simulink model "Model_FC_v4"  (R2015a)
settings: Solver=ode3  StartTime=0.0  StopTime=50  FixedStep=0.01  RelTol=1e-3
undefined symbols (not defined in the file): sigbuilder_block
libraries: powerlib x5, simulink x2
settings Model: Creator=Mina  LastModifiedBy=Mina
settings OptimizationCC: BlockReduction=off  ConditionallyExecuteInputs=off

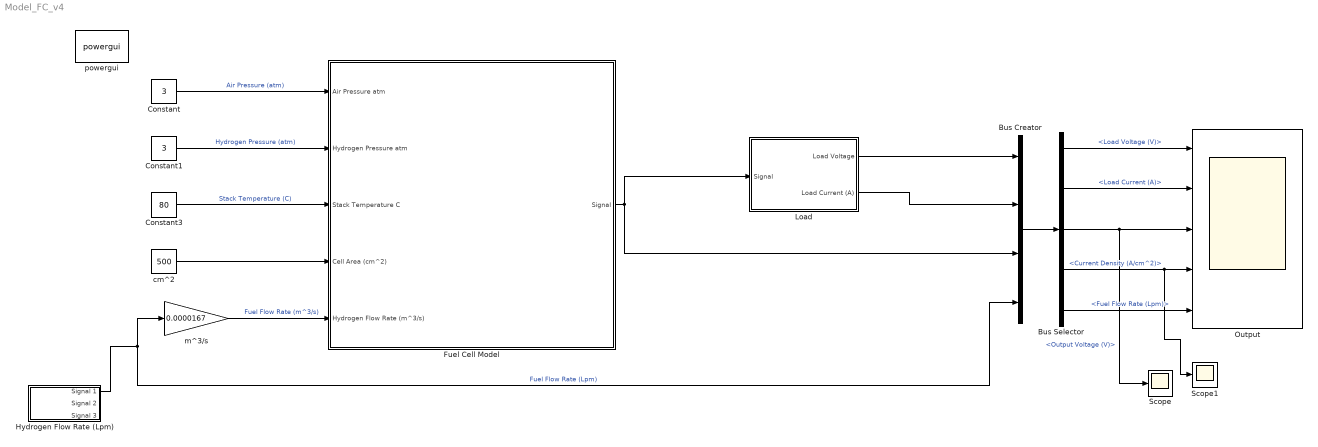
== system Model_FC_v4 ==
  Bus Creator : BusCreator
  Bus Selector : BusSelector  OutputSignals=Load Voltage (V),Load Current (A),signal3.Output Voltage (V),signal3.Current Density (A/cm^2),Fuel Flow Rate (Lpm)
  Constant : Constant  Value=3
  Constant1 : Constant  Value=3
  Constant3 : Constant  Value=80
  Fuel Cell Model : Subsystem
  Hydrogen Flow Rate (Lpm) : Subsystem  Tag=STV Subsys  LoadFcn=sigbuilder_block('load');  StartFcn=sigbuilder_block('start');  StopFcn=sigbuilder_block('stop');  ClipboardFcn=sigbuilder_block('clipboard');  mask(Sigbuilder block){}
      mask help: Simulink:masks:SigbuilderBlock_MD
      mask init:
      | if ~strcmp(get_param(bdroot(gcbh),'SimulationStatus'),'stopped') tuvar = sigbuilder_block('maskInit'); end
      settings: CopyFcn=sigbuilder_block('copy');  DeleteFcn=sigbuilder_block('delete');  ModelCloseFcn=sigbuilder_block('modelClose');  PreSaveFcn=sigbuilder_block('preSave');  PauseFcn=sigbuilder_block('pause');  ContinueFcn=sigbuilder_block('continue');  NameChangeFcn=sigbuilder_block('namechange');  OpenFcn=sigbuilder_block('open',[437.6 199.2 550.4 400 ]);  CloseFcn=sigbuilder_block('close');
      mask Display: plot(0, 0, 100, 100,[2, 2, 32, 32, 2], [68, 8, 8, 68, 68],[32, 2], [38, 38], [32, 19, 2],[53, 60, 44], [32, 17, 17, 2],[16, 16, 31, 31]);txt = getActiveGroup(gcbh);text(2, 100, txt,'verticalAlignment', 'top');
  Load : Subsystem
  "Output " : Scope  NumInputPorts=5
      settings: YMin=6~0.3~0.4~0.8~2.5  YMax=11~0.575~0.8~1.35~4  SaveName=Output_Data
  Scope : Scope
      settings: YMin=0.433555  YMax=0.433555  SaveName=ScopeData3
  Scope1 : Scope
      settings: YMin=1.24134  YMax=1.372  SaveName=ScopeData4
  cm^2 : Constant  Value=500
  m^3/s : Gain  Gain=0.0000167
  powergui : powerlib/powergui  Priority=1  SimulationMode=Continuous  SolverType=Tustin/Backward Euler (TBE)  SampleTime=50e-6  frequency=60  SPID=off  DisableSnubberDevices=off  DisableRonSwitches=off  DisableVfSwitches=off  SwTol=0  DisplayEquations=off  Interpol=off  methode=off  Ts=100  FunctionMessages=off  echomessages=off  HookPort=off  EnableUseOfTLC=off  x0status=blocks  frequencyindice=0  Pbase=100e6  ErrMax=1e-4  Iterations=50  UnitsV=kV  UnitsW=MW  buscounter=0  RestoreLinks=warning  ResistiveCurrentMeasurement=off  Frange=[0:2:500]  Ylog=off  Xlog=on  ShowGrid=off  save=off  variable=ZData  structure=0  ZoomFFT=off  StartTime=0.0  cycles=1  DisplayStyle=1  fundamental=60  FreqAxis=off  MaxFrequency=1000  frequencyindicesteady=1  RmsSteady=1  display=off
  wires:
  Constant3/1 -> Fuel Cell Model/3(Stack Temperature C)  "Stack Temperature (C)"
  cm^2/1 -> Fuel Cell Model/4(Cell Area (cm^2))
  Constant/1 -> Fuel Cell Model/1(Air Pressure atm)  "Air Pressure (atm)"
  Bus Creator/1 -> Bus Selector/1
  Bus Selector/1 -> "Output "/1  "<Load Voltage (V)>"
  Bus Selector/2 -> "Output "/2  "<Load Current (A)>"
  Bus Selector/4 -> Scope1/1, "Output "/4  "<Current Density (A/cm^2)>"
  Constant1/1 -> Fuel Cell Model/2(Hydrogen Pressure atm)  "Hydrogen Pressure (atm)"
  m^3/s/1 -> Fuel Cell Model/5(Hydrogen Flow Rate (m^3/s))  "Fuel Flow Rate (m^3/s)"
  Fuel Cell Model/1(Signal) -> Load/1(Signal), Bus Creator/3
  Bus Selector/3 -> Scope/1, "Output "/3  "<Output Voltage (V)>"
  Load/2(Load Current (A)) -> Bus Creator/2
  Load/1(Load Voltage) -> Bus Creator/1
  Hydrogen Flow Rate (Lpm)/1(Signal 1) -> Bus Creator/4, m^3/s/1  "Fuel Flow Rate (Lpm)"
  Bus Selector/5 -> "Output "/5  "<Fuel Flow Rate (Lpm)>"

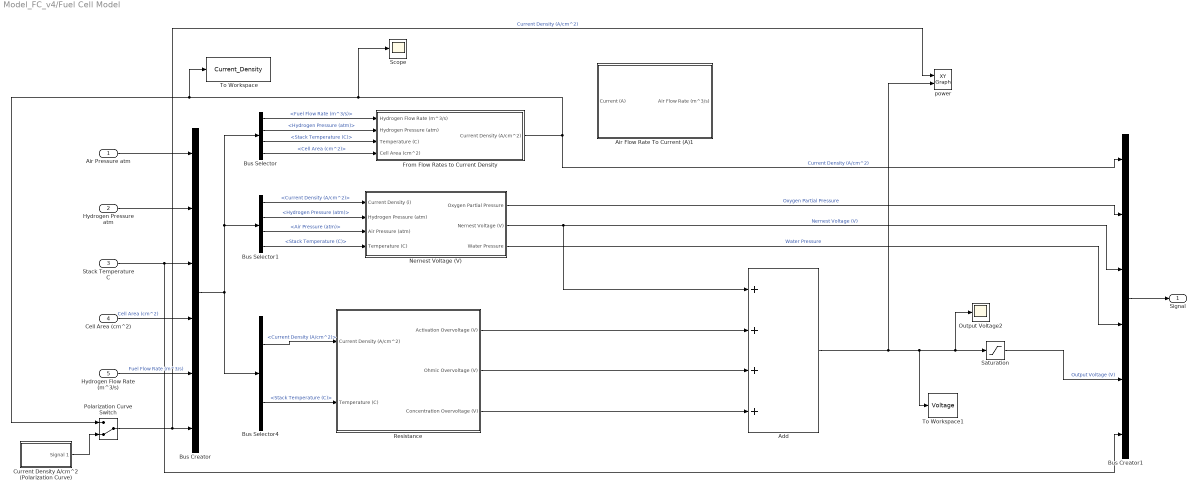
== system Model_FC_v4/Fuel Cell Model ==
  Air Pressure atm : Inport
  Hydrogen Pressure atm : Inport  Port=2
  Stack Temperature C : Inport  Port=3
  Cell Area (cm^2) : Inport  Port=4
  Hydrogen Flow Rate (m^3/s) : Inport  Port=5
  Add : Sum  Inputs=++++
  Air Flow Rate To Current (A)1 : Subsystem
  Bus Creator : BusCreator  Inputs=6
  Bus Creator1 : BusCreator  Inputs=6
  Bus Selector : BusSelector  OutputSignals=Fuel Flow Rate (m^3/s),Hydrogen Pressure (atm),Stack Temperature (C),Cell Area (cm^2)
  Bus Selector1 : BusSelector  OutputSignals=Current Density (A/cm^2),Hydrogen Pressure (atm),Air Pressure (atm),Stack Temperature (C)
  Bus Selector4 : BusSelector  OutputSignals=Current Density (A/cm^2),Stack Temperature (C)
  Current Density A/cm^2 (Polarization Curve) : Subsystem  Tag=STV Subsys  LoadFcn=sigbuilder_block('load');  StartFcn=sigbuilder_block('start');  StopFcn=sigbuilder_block('stop');  ClipboardFcn=sigbuilder_block('clipboard');  mask(Sigbuilder block){}
      mask help: Simulink:masks:SigbuilderBlock_MD
      mask init:
      | if ~strcmp(get_param(bdroot(gcbh),'SimulationStatus'),'stopped') tuvar = sigbuilder_block('maskInit'); end
      settings: CopyFcn=sigbuilder_block('copy');  DeleteFcn=sigbuilder_block('delete');  ModelCloseFcn=sigbuilder_block('modelClose');  PreSaveFcn=sigbuilder_block('preSave');  PauseFcn=sigbuilder_block('pause');  ContinueFcn=sigbuilder_block('continue');  NameChangeFcn=sigbuilder_block('namechange');  OpenFcn=sigbuilder_block('open',[437.6 199.2 550.4 400 ]);  CloseFcn=sigbuilder_block('close');
      mask Display: plot(0, 0, 100, 100,[2, 2, 32, 32, 2], [68, 8, 8, 68, 68],[32, 2], [38, 38], [32, 19, 2],[53, 60, 44], [32, 17, 17, 2],[16, 16, 31, 31]);txt = getActiveGroup(gcbh);text(2, 100, txt,'verticalAlignment', 'top');
  From Flow Rates to Current Density : Subsystem
  Nernest Voltage (V) : Subsystem
  Output Voltage2 : Scope
      settings: YMin=0.941209  YMax=0.941209  Decimation=2
  Polarization Curve Switch : ManualSwitch  CurrentSetting=0
  Resistance : Subsystem
  Saturation : Saturate  UpperLimit=inf  LowerLimit=0
  Scope : Scope
      settings: YMin=1.63334  YMax=1.63334
  To Workspace : ToWorkspace  VariableName=Current_Density  SampleTime=-1
      settings: Save2DSignal=2-D array (concatenate along first dimension)
  To Workspace1 : ToWorkspace  VariableName=Voltage  SampleTime=-1
      settings: Save2DSignal=2-D array (concatenate along first dimension)
  power : simulink/Sinks/XY Graph  xmin=0  xmax=1.5  ymin=0.0  ymax=1.4  st=0
  Signal : Outport
  wires:
  Add/1 -> power/2, To Workspace1/1, Output Voltage2/1, Saturation/1
  Cell Area (cm^2)/1 -> Bus Creator/4  "Cell Area (cm^2)"
  Saturation/1 -> Bus Creator1/5  "Output Voltage (V)"
  Current Density A/cm^2 (Polarization Curve)/1(Signal 1) -> Polarization Curve Switch/2
  Air Pressure atm/1 -> Bus Creator/1
  Hydrogen Pressure atm/1 -> Bus Creator/2
  Stack Temperature C/1 -> Bus Creator1/6, Bus Creator/3
  Hydrogen Flow Rate (m^3/s)/1 -> Bus Creator/5  "Fuel Flow Rate (m^3/s)"
  Bus Creator/1 -> Bus Selector1/1, Bus Selector/1, Bus Selector4/1
  From Flow Rates to Current Density/1(Current Density (A/cm^2)) -> Scope/1, To Workspace/1, Polarization Curve Switch/1, Bus Creator1/1  "Current Density (A/cm^2)"
  Bus Selector/1 -> From Flow Rates to Current Density/1(Hydrogen Flow Rate (m^3/s))  "<Fuel Flow Rate (m^3/s)>"
  Bus Selector/2 -> From Flow Rates to Current Density/2(Hydrogen Pressure (atm))  "<Hydrogen Pressure (atm)>"
  Bus Selector/3 -> From Flow Rates to Current Density/3(Temperature (C))  "<Stack Temperature (C)>"
  Bus Selector/4 -> From Flow Rates to Current Density/4(Cell Area (cm^2))  "<Cell Area (cm^2)>"
  Nernest Voltage (V)/2(Nernest Voltage (V)) -> Bus Creator1/3, Add/1  "Nernest Voltage (V)"
  Bus Selector1/1 -> Nernest Voltage (V)/1(Current Density (i))  "<Current Density (A/cm^2)>"
  Bus Selector1/2 -> Nernest Voltage (V)/2(Hydrogen Pressure (atm))  "<Hydrogen Pressure (atm)>"
  Bus Selector1/3 -> Nernest Voltage (V)/3(Air Pressure (atm))  "<Air Pressure (atm)>"
  Bus Selector1/4 -> Nernest Voltage (V)/4(Temperature (C))  "<Stack Temperature (C)>"
  Nernest Voltage (V)/1(Oxygen Partial Pressure) -> Bus Creator1/2  "Oxygen Partial Pressure"
  Nernest Voltage (V)/3(Water Pressure) -> Bus Creator1/4  "Water Pressure"
  Bus Selector4/1 -> Resistance/1(Current Density (A/cm^2))  "<Current Density (A/cm^2)>"
  Bus Selector4/2 -> Resistance/2(Temperature (C))  "<Stack Temperature (C)>"
  Resistance/1(Activation Overvoltage (V)) -> Add/2
  Resistance/2(Ohmic Overvoltage (V)) -> Add/3
  Resistance/3(Concentration Overvoltage (V)) -> Add/4
  Polarization Curve Switch/1 -> power/1, Bus Creator/6  "Current Density (A/cm^2)"
  Bus Creator1/1 -> Signal/1

== system Model_FC_v4/Hydrogen Flow Rate (Lpm) ==
  Demux : Demux  Tag=STV Demux  Outputs=3
  FromWs : FromWorkspace  Tag=STV FromWs  VariableName=tuvar  SampleTime=0
      SigBuilderData=|
      | common.afterFinalStr = 'Extrapolate'
      | common.sampleTime = 0
      | dataSet.timeRange = [0 10]
      | dataSet.name = 'Group 1'
      | sbobj.Groups.Name = 'Group 1'
      | sbobj.Groups.Signals(1).Name = 'Signal 1'
      | sbobj.Groups.Signals(1).XData = [0 5 7.5 10]
      | sbobj.Groups.Signals(1).YData = [2.5 2.5 4 4]
      | sbobj.Groups.Signals(2).Name = 'Signal 2'
      | sbobj.Groups.Signals(2).XData = [0 5 5 10]
      | sbobj.Groups.Signals(2).YData = [2.5 2.5 4 4]
      | sbobj.Groups.Signals(3).Name = 'Signal 3'
      | sbobj.Groups.Signals(3).XData = [0 10]
      | sbobj.Groups.Signals(3).YData = [4 4]
  Signal 1 : Outport  Tag=STV Outport
  Signal 2 : Outport  Tag=STV Outport  Port=2
  Signal 3 : Outport  Tag=STV Outport  Port=3
  wires:
  Demux/1 -> Signal 1/1
  FromWs/1 -> Demux/1
  Demux/2 -> Signal 2/1
  Demux/3 -> Signal 3/1

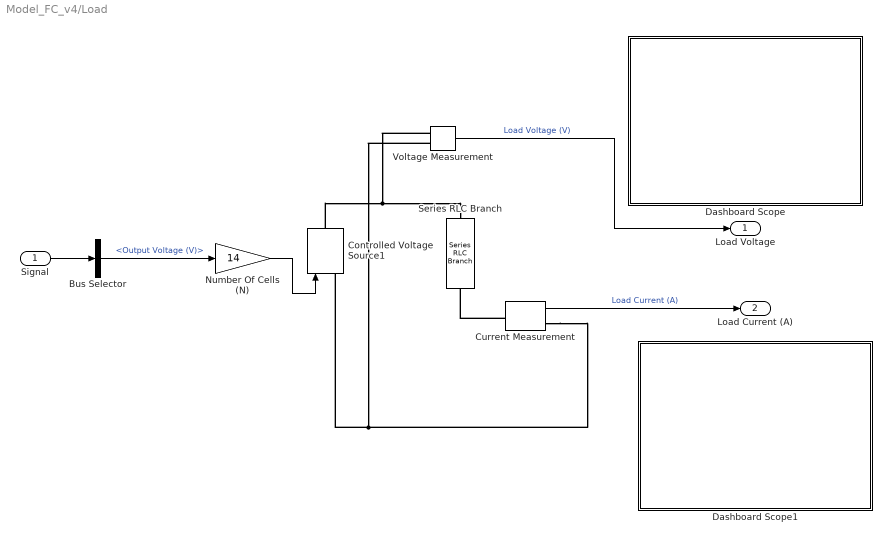
== system Model_FC_v4/Load ==
  Signal : Inport
  Bus Selector : BusSelector  OutputSignals=Output Voltage (V)
  Controlled Voltage Source1 : powerlib/Electrical Sources/Controlled Voltage Source  Initialize=on  Source_Type=AC  Amplitude=0  Phase=0  Frequency=0  Measurements=None
  Current Measurement : powerlib/Measurements/Current Measurement  PhasorSimulation=off  OutputType=Complex  PSBequivalent=0
  Dashboard Scope : Subsystem  DialogController=hmiCreateDDGDialog  IsWebBlock=on  mask(MathWorksWebBlock){webBlockId=81580c46-4ac5-4980-a5b4-9a4d2062d879, webBlockType=sdiscope, ShowInitialText=on, HMISrcModelName=Model_FC_v4}
      mask prompts: webBlockId "WebBlock Id"; webBlockType "WebBlock Type"; HMISrcModelName "Source Model"
      mask Help: helpview([docroot '/mapfiles/simulink.map'], 'hmi_scope')
      mask Display:
      | if strcmp(get_param(bdroot(gcb),'BlockDiagramType'), 'library')
      |     image([(matlabroot) '/toolbox/simulink/hmi/icons/DashboardScope.png']);
      | end
  Dashboard Scope1 : Subsystem  DialogController=hmiCreateDDGDialog  IsWebBlock=on  mask(MathWorksWebBlock){webBlockId=c4e3daab-8dab-4642-a272-c974aaedb1ac, webBlockType=sdiscope, ShowInitialText=on, HMISrcModelName=Model_FC_v4}
      mask prompts: webBlockId "WebBlock Id"; webBlockType "WebBlock Type"; HMISrcModelName "Source Model"
      mask Help: helpview([docroot '/mapfiles/simulink.map'], 'hmi_scope')
      mask Display:
      | if strcmp(get_param(bdroot(gcb),'BlockDiagramType'), 'library')
      |     image([(matlabroot) '/toolbox/simulink/hmi/icons/DashboardScope.png']);
      | end
  Number Of Cells (N) : Gain  Gain=14
  Series RLC Branch : powerlib/Elements/Series RLC Branch  LConnTagsString=__new0  RConnTagsString=__new0  BranchType=R  Resistance=19.36  Inductance=100*100/6000  SetiL0=off  InitialCurrent=0  Capacitance=1e-6  Setx0=off  InitialVoltage=0  Measurements=None
  Voltage Measurement : powerlib/Measurements/Voltage Measurement  PhasorSimulation=off  OutputType=Complex  PSBequivalent=0
  Load Voltage : Outport
  Load Current (A) : Outport  Port=2
  wires:
  Current Measurement/1 -> Load Current (A)/1  "Load Current (A)"
  Voltage Measurement/1 -> Load Voltage/1  "Load Voltage (V)"
  Number Of Cells (N)/1 -> Controlled Voltage Source1/1
  Signal/1 -> Bus Selector/1
  Bus Selector/1 -> Number Of Cells (N)/1  "<Output Voltage (V)>"
  connections:
  Controlled Voltage Source1/RConn1 -- Voltage Measurement/LConn1 -- Series RLC Branch/LConn1
  Current Measurement/LConn1 -- Series RLC Branch/RConn1
  Current Measurement/RConn1 -- Voltage Measurement/LConn2 -- Controlled Voltage Source1/LConn1

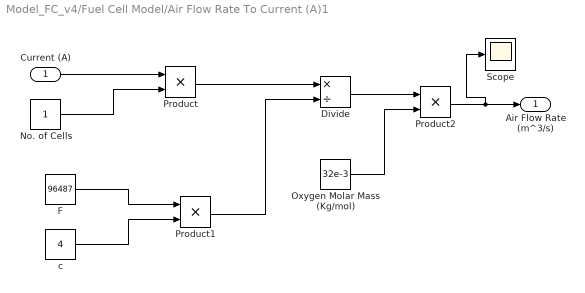
== system Model_FC_v4/Fuel Cell Model/Air Flow Rate To Current (A)1 ==
  Current (A) : Inport
  Divide : Product  Inputs=*/
  F : Constant  Value=96487
  No. of Cells : Constant
  Oxygen Molar Mass (Kg/mol) : Constant  Value=32e-3
  Product : Product
  Product1 : Product
  Product2 : Product
  Scope : Scope
      settings: SaveName=ScopeData7
  c : Constant  Value=4
  Air Flow Rate (m^3/s) : Outport
  wires:
  Current (A)/1 -> Product/1
  No. of Cells/1 -> Product/2
  Product/1 -> Divide/1
  F/1 -> Product1/1
  c/1 -> Product1/2
  Product1/1 -> Divide/2
  Divide/1 -> Product2/1
  Oxygen Molar Mass (Kg/mol)/1 -> Product2/2
  Product2/1 -> Scope/1, Air Flow Rate (m^3/s)/1

== system Model_FC_v4/Fuel Cell Model/Current Density A//cm^2 (Polarization Curve) ==
  Demux : Demux  Tag=STV Demux  Outputs=1
  FromWs : FromWorkspace  Tag=STV FromWs  VariableName=tuvar  SampleTime=0
      SigBuilderData=|
      | common.afterFinalStr = 'Extrapolate'
      | common.sampleTime = 0
      | dataSet.timeRange = [0 10]
      | dataSet.name = 'Group 1'
      | sbobj.Groups.Name = 'Group 1'
      | sbobj.Groups.Signals.Name = 'Signal 1'
      | sbobj.Groups.Signals.XData = [0 2.5 5 10]
      | sbobj.Groups.Signals.YData = [0.01 0.7 1.39 1.39]
  Signal 1 : Outport  Tag=STV Outport
  wires:
  Demux/1 -> Signal 1/1
  FromWs/1 -> Demux/1

== system Model_FC_v4/Fuel Cell Model/From Flow Rates to Current Density ==
  Hydrogen Flow Rate (m^3/s) : Inport
  Hydrogen Pressure (atm) : Inport  Port=2
  Temperature (C) : Inport  Port=3
  Cell Area (cm^2) : Inport  Port=4
  Fuel Flow Rate To Current (A) : Subsystem
  Subsystem1 : Subsystem
  Current Density (A/cm^2) : Outport
  wires:
  Cell Area (cm^2)/1 -> Subsystem1/2(Cell Area (cm^2))
  Fuel Flow Rate To Current (A)/1(Current (A)) -> Subsystem1/1(Nominal Current (A))
  Hydrogen Flow Rate (m^3/s)/1 -> Fuel Flow Rate To Current (A)/1(Hydrogen Flow Rate (m^3/s))
  Hydrogen Pressure (atm)/1 -> Fuel Flow Rate To Current (A)/2(Hydrogen Pressure (atm))
  Temperature (C)/1 -> Fuel Flow Rate To Current (A)/3(T (C))
  Subsystem1/1(Current Density (A/cm^2)) -> Current Density (A/cm^2)/1  "Current density (A/cm^2)"

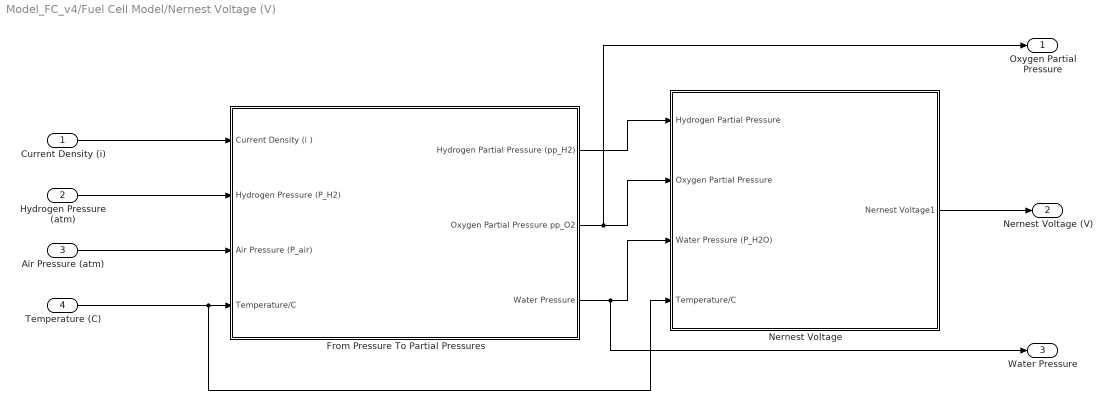
== system Model_FC_v4/Fuel Cell Model/Nernest Voltage (V) ==
  Current Density (i) : Inport
  Hydrogen Pressure (atm) : Inport  Port=2
  Air Pressure (atm) : Inport  Port=3
  Temperature (C) : Inport  Port=4
  From Pressure To Partial Pressures : Subsystem
  Nernest Voltage : Subsystem
  Oxygen Partial Pressure : Outport
  Nernest Voltage (V) : Outport  Port=2
  Water Pressure : Outport  Port=3
  wires:
  Temperature (C)/1 -> Nernest Voltage/4(Temperature/C), From Pressure To Partial Pressures/4(Temperature/C)
  From Pressure To Partial Pressures/1(Hydrogen Partial Pressure (pp_H2)) -> Nernest Voltage/1(Hydrogen Partial Pressure)
  Hydrogen Pressure (atm)/1 -> From Pressure To Partial Pressures/2(Hydrogen Pressure (P_H2))
  Nernest Voltage/1(Nernest Voltage1) -> Nernest Voltage (V)/1
  From Pressure To Partial Pressures/2(Oxygen Partial Pressure pp_O2) -> Oxygen Partial Pressure/1, Nernest Voltage/2(Oxygen Partial Pressure)
  From Pressure To Partial Pressures/3(Water Pressure) -> Water Pressure/1, Nernest Voltage/3(Water Pressure (P_H2O))
  Current Density (i)/1 -> From Pressure To Partial Pressures/1(Current Density (i ))
  Air Pressure (atm)/1 -> From Pressure To Partial Pressures/3(Air Pressure (P_air))

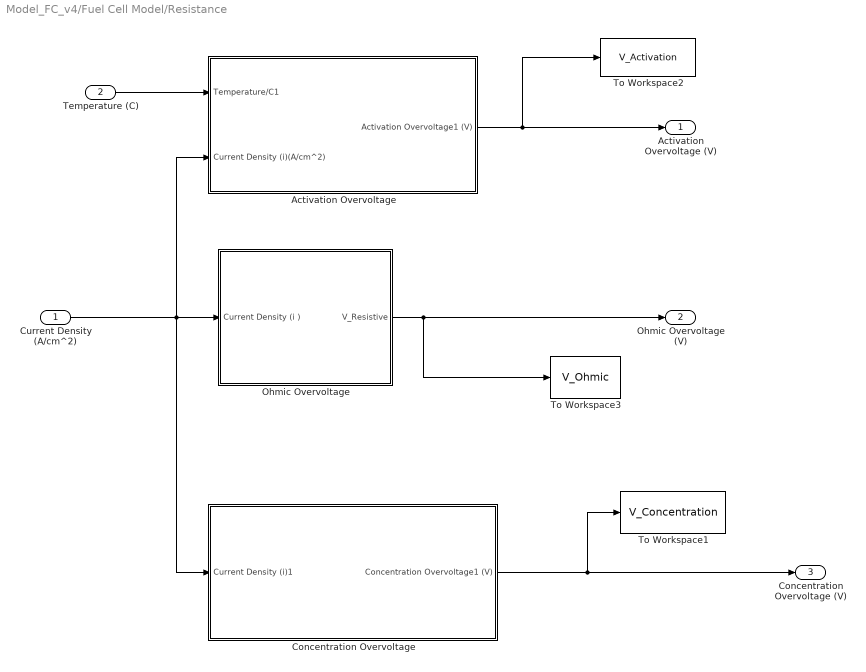
== system Model_FC_v4/Fuel Cell Model/Resistance ==
  Current Density (A/cm^2) : Inport
  Temperature (C) : Inport  Port=2
  Activation Overvoltage : Subsystem
  Concentration Overvoltage : Subsystem
  Ohmic Overvoltage : Subsystem
  To Workspace1 : ToWorkspace  VariableName=V_Concentration  SampleTime=-1
      settings: Save2DSignal=2-D array (concatenate along first dimension)
  To Workspace2 : ToWorkspace  VariableName=V_Activation  SampleTime=-1
      settings: Save2DSignal=2-D array (concatenate along first dimension)
  To Workspace3 : ToWorkspace  VariableName=V_Ohmic  SampleTime=-1
      settings: Save2DSignal=2-D array (concatenate along first dimension)
  Activation Overvoltage (V) : Outport
  Ohmic Overvoltage (V) : Outport  Port=2
  Concentration Overvoltage (V) : Outport  Port=3
  wires:
  Temperature (C)/1 -> Activation Overvoltage/1(Temperature/C1)
  Current Density (A/cm^2)/1 -> Activation Overvoltage/2(Current Density (i)(A/cm^2)), Concentration Overvoltage/1(Current Density (i)1), Ohmic Overvoltage/1(Current Density (i ))
  Ohmic Overvoltage/1(V_Resistive) -> Ohmic Overvoltage (V)/1, To Workspace3/1
  Activation Overvoltage/1(Activation Overvoltage1 (V)) -> To Workspace2/1, Activation Overvoltage (V)/1
  Concentration Overvoltage/1("Concentration Overvoltage1 (V) ") -> To Workspace1/1, Concentration Overvoltage (V)/1

== system Model_FC_v4/Load/Dashboard Scope ==

== system Model_FC_v4/Load/Dashboard Scope1 ==

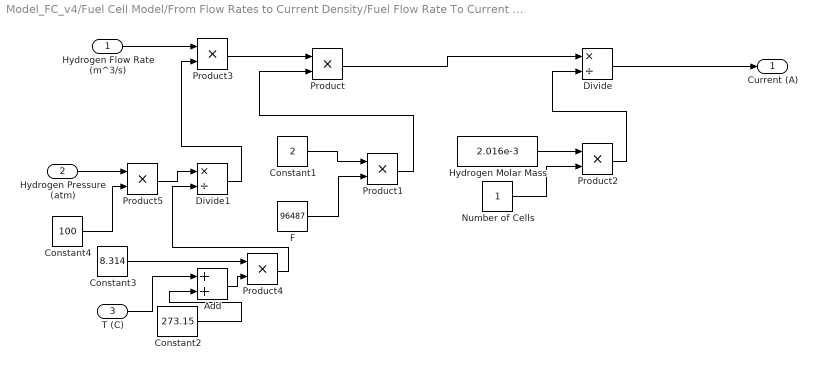
== system Model_FC_v4/Fuel Cell Model/From Flow Rates to Current Density/Fuel Flow Rate To Current (A) ==
  Hydrogen Flow Rate (m^3/s) : Inport
  Hydrogen Pressure (atm) : Inport  Port=2
  T (C) : Inport  Port=3
  Add : Sum
  Constant1 : Constant  Value=2
  Constant2 : Constant  Value=273.15
  Constant3 : Constant  Value=8.314
  Constant4 : Constant  Value=100
  Divide : Product  Inputs=*/
  Divide1 : Product  Inputs=*/
  F : Constant  Value=96487
  Hydrogen Molar Mass : Constant  Value=2.016e-3
  Number of Cells : Constant
  Product{,1..5} (6 alike) : Product
  Current (A) : Outport
  wires:
  Hydrogen Flow Rate (m^3/s)/1 -> Product3/1
  F/1 -> Product1/2
  Constant1/1 -> Product1/1
  Product1/1 -> Product/2
  Product/1 -> Divide/1
  Hydrogen Molar Mass/1 -> Product2/1
  Number of Cells/1 -> Product2/2
  Product2/1 -> Divide/2
  Divide/1 -> Current (A)/1
  Hydrogen Pressure (atm)/1 -> Product5/1
  Constant3/1 -> Product4/1
  T (C)/1 -> Add/1
  Product4/1 -> Divide1/2
  Divide1/1 -> Product3/2
  Product3/1 -> Product/1
  Add/1 -> Product4/2
  Constant2/1 -> Add/2
  Constant4/1 -> Product5/2
  Product5/1 -> Divide1/1

== system Model_FC_v4/Fuel Cell Model/From Flow Rates to Current Density/Subsystem1 ==
  Nominal Current (A) : Inport
  Cell Area (cm^2) : Inport  Port=2
  Divide : Product  Inputs=*/
  Current Density (A/cm^2) : Outport
  wires:
  Nominal Current (A)/1 -> Divide/1
  Cell Area (cm^2)/1 -> Divide/2
  Divide/1 -> Current Density (A/cm^2)/1

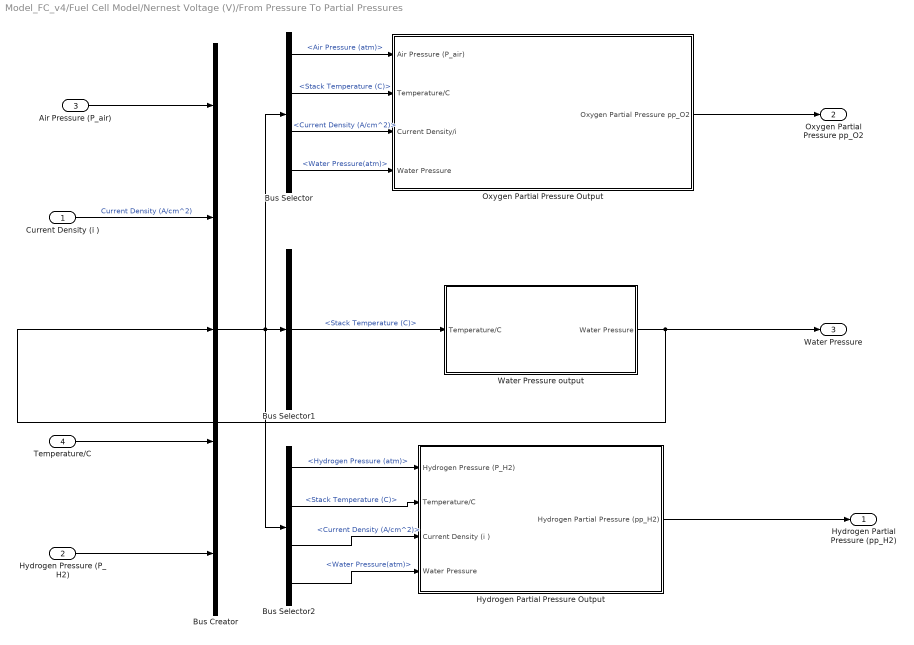
== system Model_FC_v4/Fuel Cell Model/Nernest Voltage (V)/From Pressure To Partial Pressures ==
  Current Density (i ) : Inport
  Hydrogen Pressure (P_H2) : Inport  Port=2
  Air Pressure (P_air) : Inport  Port=3
  Temperature/C : Inport  Port=4
  Bus Creator : BusCreator  Inputs=5
  Bus Selector : BusSelector  OutputSignals=Air Pressure (atm),Stack Temperature (C),Current Density (A/cm^2),Water Pressure(atm)
  Bus Selector1 : BusSelector  OutputSignals=Stack Temperature (C)
  Bus Selector2 : BusSelector  OutputSignals=Hydrogen Pressure (atm),Stack Temperature (C),Current Density (A/cm^2),Water Pressure(atm)
  Hydrogen Partial Pressure Output : Subsystem
  Oxygen Partial Pressure Output : Subsystem
  Water Pressure output : Subsystem
  Hydrogen Partial Pressure (pp_H2) : Outport
  Oxygen Partial Pressure pp_O2 : Outport  Port=2
  Water Pressure : Outport  Port=3
  wires:
  Water Pressure output/1(Water Pressure) -> Water Pressure/1, Bus Creator/3
  Air Pressure (P_air)/1 -> Bus Creator/1
  Oxygen Partial Pressure Output/1(Oxygen Partial Pressure pp_O2) -> Oxygen Partial Pressure pp_O2/1
  Hydrogen Partial Pressure Output/1(Hydrogen Partial Pressure (pp_H2)) -> Hydrogen Partial Pressure (pp_H2)/1
  Current Density (i )/1 -> Bus Creator/2  "Current Density (A/cm^2)"
  Temperature/C/1 -> Bus Creator/4
  Hydrogen Pressure (P_H2)/1 -> Bus Creator/5
  Bus Creator/1 -> Bus Selector2/1, Bus Selector/1, Bus Selector1/1
  Bus Selector/1 -> Oxygen Partial Pressure Output/1(Air Pressure (P_air))  "<Air Pressure (atm)>"
  Bus Selector/2 -> Oxygen Partial Pressure Output/2(Temperature/C)  "<Stack Temperature (C)>"
  Bus Selector/3 -> Oxygen Partial Pressure Output/3(Current Density/i)  "<Current Density (A/cm^2)>"
  Bus Selector/4 -> Oxygen Partial Pressure Output/4(Water Pressure)  "<Water Pressure(atm)>"
  Bus Selector1/1 -> Water Pressure output/1(Temperature/C)  "<Stack Temperature (C)>"
  Bus Selector2/1 -> Hydrogen Partial Pressure Output/1(Hydrogen Pressure (P_H2))  "<Hydrogen Pressure (atm)>"
  Bus Selector2/2 -> Hydrogen Partial Pressure Output/2(Temperature/C)  "<Stack Temperature (C)>"
  Bus Selector2/3 -> Hydrogen Partial Pressure Output/3(Current Density (i ))  "<Current Density (A/cm^2)>"
  Bus Selector2/4 -> Hydrogen Partial Pressure Output/4(Water Pressure)  "<Water Pressure(atm)>"

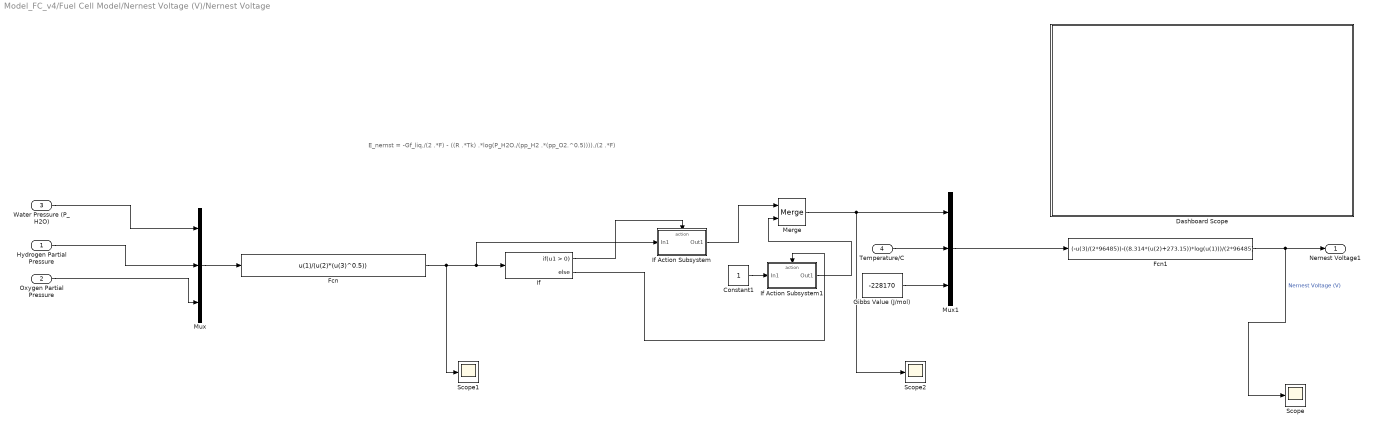
== system Model_FC_v4/Fuel Cell Model/Nernest Voltage (V)/Nernest Voltage ==
  note: E_nernst = -Gf_liq./(2 .*F) - ((R .*Tk) .*log(P_H2O./(pp_H2 .*(pp_O2.^0.5))))./(2 .*F)
  Hydrogen Partial Pressure : Inport
  Oxygen Partial Pressure : Inport  Port=2
  Water Pressure (P_H2O) : Inport  Port=3
  Temperature/C : Inport  Port=4
  Constant1 : Constant
  Dashboard Scope : Subsystem  DialogController=hmiCreateDDGDialog  IsWebBlock=on  mask(MathWorksWebBlock){webBlockId=5bd8e11a-4211-42d2-b432-bf660f2594da, webBlockType=sdiscope, ShowInitialText=on, HMISrcModelName=Model_FC_v4}
      mask prompts: webBlockId "WebBlock Id"; webBlockType "WebBlock Type"; HMISrcModelName "Source Model"
      mask Help: helpview([docroot '/mapfiles/simulink.map'], 'hmi_scope')
      mask Display:
      | if strcmp(get_param(bdroot(gcb),'BlockDiagramType'), 'library')
      |     image([(matlabroot) '/toolbox/simulink/hmi/icons/DashboardScope.png']);
      | end
  Fcn : Fcn  Expr=u(1)/(u(2)*(u(3)^0.5))
  Fcn1 : Fcn  Expr=(-u(3)/(2*96485))-((8.314*(u(2)+273.15))*log(u(1)))/(2*96485)
  Gibbs Value (J/mol) : Constant  Value=-228170
  If : If
  If Action Subsystem : Subsystem  TreatAsAtomicUnit=on
  If Action Subsystem1 : Subsystem  TreatAsAtomicUnit=on
  Merge : Merge
  Mux : Mux  Inputs=3
  Mux1 : Mux  Inputs=3
  Scope : Scope
      settings: YMin=1.18241  YMax=1.18241  SaveName=ScopeData13
  Scope1 : Scope
      settings: YMin=35118.6  YMax=38815.2  SaveName=ScopeData14
  Scope2 : Scope
      settings: YMin=35118.6  YMax=38815.2  SaveName=ScopeData15
  Nernest Voltage1 : Outport
  wires:
  Gibbs Value (J/mol)/1 -> Mux1/3
  Oxygen Partial Pressure/1 -> Mux/3
  If/1 -> If Action Subsystem/Action
  If Action Subsystem/1(Out1) -> Merge/1
  If/2 -> If Action Subsystem1/Action
  Constant1/1 -> If Action Subsystem1/1(In1)
  If Action Subsystem1/1(Out1) -> Merge/2
  Water Pressure (P_H2O)/1 -> Mux/1
  Hydrogen Partial Pressure/1 -> Mux/2
  Mux/1 -> Fcn/1
  Fcn/1 -> Scope1/1, If Action Subsystem/1(In1), If/1
  Merge/1 -> Scope2/1, Mux1/1
  Temperature/C/1 -> Mux1/2
  Mux1/1 -> Fcn1/1
  Fcn1/1 -> Scope/1, Nernest Voltage1/1  "Nernest Voltage (V)"

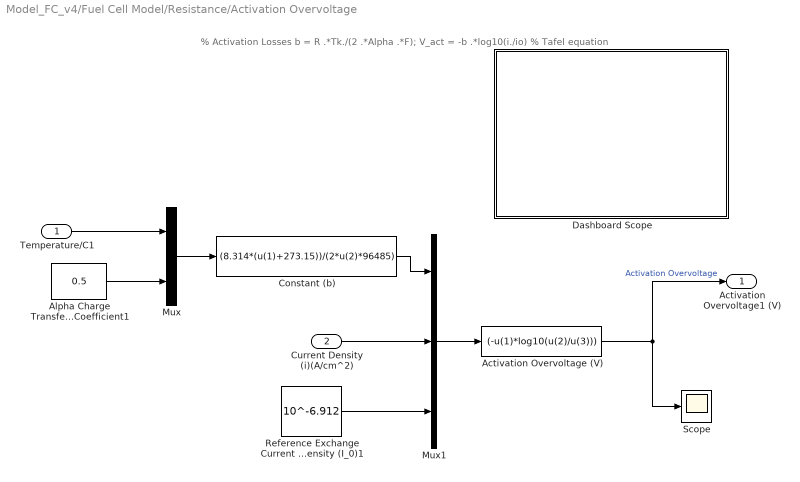
== system Model_FC_v4/Fuel Cell Model/Resistance/Activation Overvoltage ==
  note: % Activation Losses
      | b = R .*Tk./(2 .*Alpha .*F);
      | V_act = -b .*log10(i./io) % Tafel equation
  Temperature/C1 : Inport
  Current Density (i)(A/cm^2) : Inport  Port=2
  Activation Overvoltage (V) : Fcn  Expr=(-u(1)*log10(u(2)/u(3)))
  Alpha Charge Transfer Coefficient1 : Constant  Value=0.5
  Constant (b) : Fcn  Expr=(8.314*(u(1)+273.15))/(2*u(2)*96485)
  Dashboard Scope : Subsystem  DialogController=hmiCreateDDGDialog  IsWebBlock=on  mask(MathWorksWebBlock){webBlockId=22b8d2ec-b744-4464-9b72-15b4b53948fb, webBlockType=sdiscope, ShowInitialText=on, HMISrcModelName=Model_FC_v4}
      mask prompts: webBlockId "WebBlock Id"; webBlockType "WebBlock Type"; HMISrcModelName "Source Model"
      mask Help: helpview([docroot '/mapfiles/simulink.map'], 'hmi_scope')
      mask Display:
      | if strcmp(get_param(bdroot(gcb),'BlockDiagramType'), 'library')
      |     image([(matlabroot) '/toolbox/simulink/hmi/icons/DashboardScope.png']);
      | end
  Mux : Mux  Inputs=2
  Mux1 : Mux  Inputs=3
  Reference Exchange Current Density (I_0)1 : Constant  Value=10^-6.912
  Scope : Scope
      settings: SaveName=ScopeData41
  Activation Overvoltage1 (V) : Outport
  wires:
  Mux/1 -> Constant (b)/1
  Alpha Charge Transfer Coefficient1/1 -> Mux/2
  Temperature/C1/1 -> Mux/1
  Mux1/1 -> Activation Overvoltage (V)/1
  Constant (b)/1 -> Mux1/1
  Current Density (i)(A/cm^2)/1 -> Mux1/2
  Reference Exchange Current Density (I_0)1/1 -> Mux1/3
  Activation Overvoltage (V)/1 -> Activation Overvoltage1 (V)/1, Scope/1  "Activation Overvoltage"

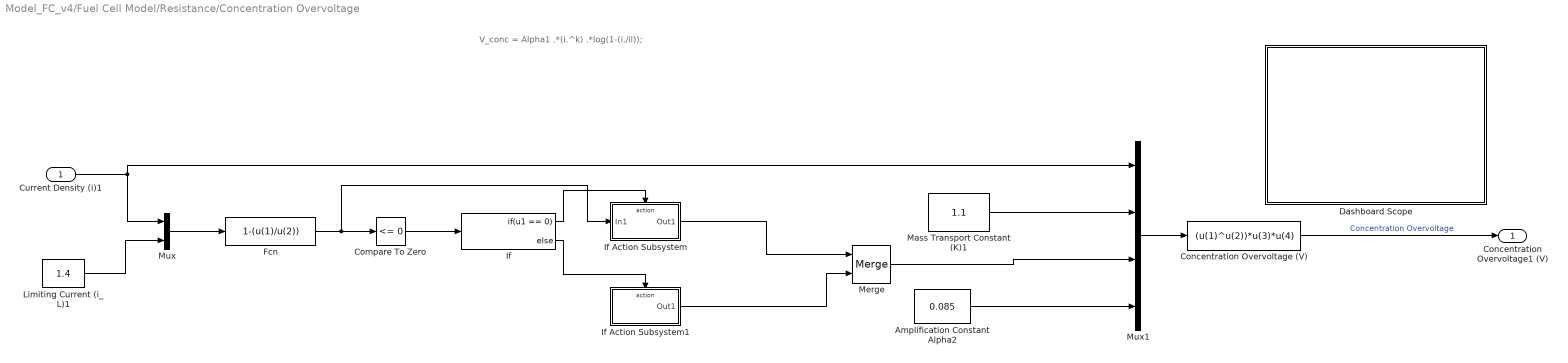
== system Model_FC_v4/Fuel Cell Model/Resistance/Concentration Overvoltage ==
  note: V_conc = Alpha1 .*(i.^k) .*log(1-(i./il));
  Current Density (i)1 : Inport
  Amplification Constant Alpha2 : Constant  Value=0.085
  Compare To Zero : simulink/Logic and Bit Operations/Compare To Zero  relop=<=  OutDataTypeStr=boolean
  Concentration Overvoltage (V) : Fcn  Expr=(u(1)^u(2))*u(3)*u(4)
  Dashboard Scope : Subsystem  DialogController=hmiCreateDDGDialog  IsWebBlock=on  mask(MathWorksWebBlock){webBlockId=564ecfdb-cb30-4ab8-9f97-8672f30b7fa2, webBlockType=sdiscope, ShowInitialText=on, HMISrcModelName=Model_FC_v4}
      mask prompts: webBlockId "WebBlock Id"; webBlockType "WebBlock Type"; HMISrcModelName "Source Model"
      mask Help: helpview([docroot '/mapfiles/simulink.map'], 'hmi_scope')
      mask Display:
      | if strcmp(get_param(bdroot(gcb),'BlockDiagramType'), 'library')
      |     image([(matlabroot) '/toolbox/simulink/hmi/icons/DashboardScope.png']);
      | end
  Fcn : Fcn  Expr=1-(u(1)/u(2))
  If : If  IfExpression=u1 == 0
  If Action Subsystem : Subsystem  TreatAsAtomicUnit=on
  If Action Subsystem1 : Subsystem  TreatAsAtomicUnit=on
  Limiting Current (i_L)1 : Constant  Value=1.4
  Mass Transport Constant (K)1 : Constant  Value=1.1
  Merge : Merge  InitialOutput=1
  Mux : Mux  Inputs=2
  Mux1 : Mux
  "Concentration Overvoltage1 (V) " : Outport
  wires:
  If/1 -> If Action Subsystem/Action
  If/2 -> If Action Subsystem1/Action
  If Action Subsystem/1(Out1) -> Merge/1
  If Action Subsystem1/1(Out1) -> Merge/2
  Compare To Zero/1 -> If/1
  Mux/1 -> Fcn/1
  Limiting Current (i_L)1/1 -> Mux/2
  Fcn/1 -> If Action Subsystem/1(In1), Compare To Zero/1
  Mux1/1 -> Concentration Overvoltage (V)/1
  Current Density (i)1/1 -> Mux1/1, Mux/1
  Mass Transport Constant (K)1/1 -> Mux1/2
  Merge/1 -> Mux1/3
  Amplification Constant Alpha2/1 -> Mux1/4
  Concentration Overvoltage (V)/1 -> "Concentration Overvoltage1 (V) "/1  "Concentration Overvoltage"

== system Model_FC_v4/Fuel Cell Model/Resistance/Ohmic Overvoltage ==
  Current Density (i ) : Inport
  Constant : Constant  Value=-1
  Dashboard Scope : Subsystem  DialogController=hmiCreateDDGDialog  IsWebBlock=on  mask(MathWorksWebBlock){webBlockId=c0b798d8-aea7-4029-a856-156eb00102c5, webBlockType=sdiscope, ShowInitialText=on, HMISrcModelName=Model_FC_v4}
      mask prompts: webBlockId "WebBlock Id"; webBlockType "WebBlock Type"; HMISrcModelName "Source Model"
      mask Help: helpview([docroot '/mapfiles/simulink.map'], 'hmi_scope')
      mask Display:
      | if strcmp(get_param(bdroot(gcb),'BlockDiagramType'), 'library')
      |     image([(matlabroot) '/toolbox/simulink/hmi/icons/DashboardScope.png']);
      | end
  Internal Resistance (r) : Constant  Value=0.19
  V_Resistive1 : Product  Inputs=3
  V_Resistive : Outport
  wires:
  Constant/1 -> V_Resistive1/3
  Internal Resistance (r)/1 -> V_Resistive1/2
  Current Density (i )/1 -> V_Resistive1/1
  V_Resistive1/1 -> V_Resistive/1  "Ohmic Overvoltage (V)"

== system Model_FC_v4/Fuel Cell Model/Nernest Voltage (V)/From Pressure To Partial Pressures/Hydrogen Partial Pressure Output ==
  note: pp_H2 = 0.5 .*((P_H2)./(exp(1.653 .*i./(Tk.^1.334)))-P_H2O)
  Hydrogen Pressure (P_H2) : Inport
  Temperature/C : Inport  Port=2
  Current Density (i ) : Inport  Port=3
  Water Pressure : Inport  Port=4
  Dashboard Scope : Subsystem  DialogController=hmiCreateDDGDialog  IsWebBlock=on  mask(MathWorksWebBlock){webBlockId=ddeef619-4d6d-4ce8-b4bd-8db147ec0074, webBlockType=sdiscope, ShowInitialText=on, HMISrcModelName=Model_FC_v4}
      mask prompts: webBlockId "WebBlock Id"; webBlockType "WebBlock Type"; HMISrcModelName "Source Model"
      mask Help: helpview([docroot '/mapfiles/simulink.map'], 'hmi_scope')
      mask Display:
      | if strcmp(get_param(bdroot(gcb),'BlockDiagramType'), 'library')
      |     image([(matlabroot) '/toolbox/simulink/hmi/icons/DashboardScope.png']);
      | end
  Fcn : Fcn  Expr=0.5*((u(1))/(exp(1.653*u(2)/((u(3)+273.15)^1.334)))-u(4))
  Mux : Mux
  Scope : Scope
      settings: SaveName=ScopeData2
  Hydrogen Partial Pressure (pp_H2) : Outport
  wires:
  Water Pressure/1 -> Mux/4
  Temperature/C/1 -> Mux/3
  Current Density (i )/1 -> Scope/1, Mux/2
  Hydrogen Pressure (P_H2)/1 -> Mux/1
  Mux/1 -> Fcn/1
  Fcn/1 -> Hydrogen Partial Pressure (pp_H2)/1  "Hydrogen Partial Pressure (pp_H2)"

== system Model_FC_v4/Fuel Cell Model/Nernest Voltage (V)/From Pressure To Partial Pressures/Oxygen Partial Pressure Output ==
  note: pp_O2 = (P_air./exp(4.192 .*i/(Tk.^1.334)))-P_H2O
  Air Pressure (P_air) : Inport
  Temperature/C : Inport  Port=2
  Current Density/i : Inport  Port=3
  Water Pressure : Inport  Port=4
  Dashboard Scope : Subsystem  DialogController=hmiCreateDDGDialog  IsWebBlock=on  mask(MathWorksWebBlock){webBlockId=99fd1843-b8cb-4f53-b690-4cde1b6230bf, webBlockType=sdiscope, ShowInitialText=on, HMISrcModelName=Model_FC_v4}
      mask prompts: webBlockId "WebBlock Id"; webBlockType "WebBlock Type"; HMISrcModelName "Source Model"
      mask Help: helpview([docroot '/mapfiles/simulink.map'], 'hmi_scope')
      mask Display:
      | if strcmp(get_param(bdroot(gcb),'BlockDiagramType'), 'library')
      |     image([(matlabroot) '/toolbox/simulink/hmi/icons/DashboardScope.png']);
      | end
  Fcn : Fcn  Expr=(u(1)/exp(4.192 *u(2)/((u(3)+273.15)^1.334)))-u(4)
  Mux : Mux
  Oxygen Partial Pressure pp_O2 : Outport
  wires:
  Current Density/i/1 -> Mux/2
  Water Pressure/1 -> Mux/4
  Temperature/C/1 -> Mux/3
  Air Pressure (P_air)/1 -> Mux/1
  Mux/1 -> Fcn/1
  Fcn/1 -> Oxygen Partial Pressure pp_O2/1  "Oxygen Partial Pressure pp_O2"

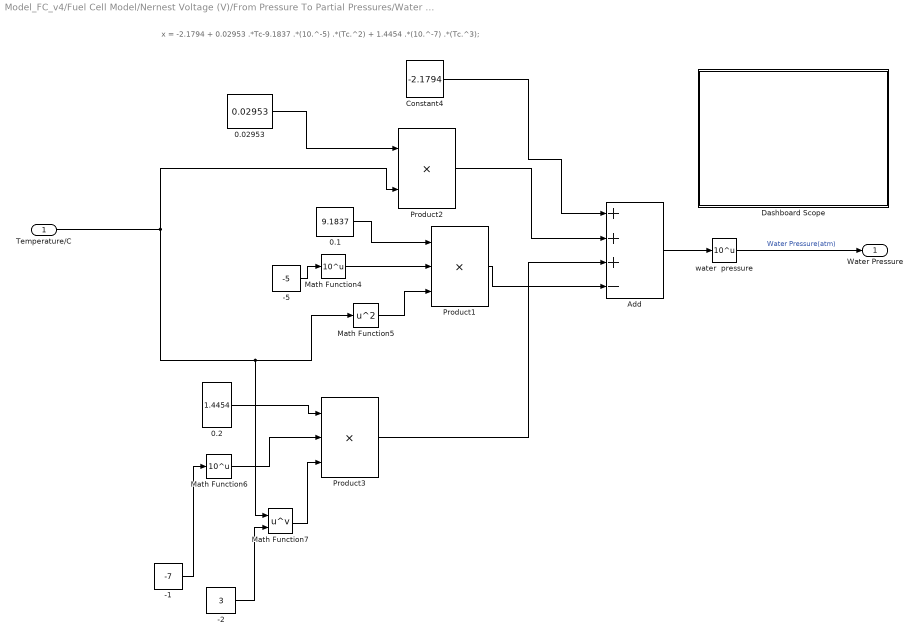
== system Model_FC_v4/Fuel Cell Model/Nernest Voltage (V)/From Pressure To Partial Pressures/Water Pressure output ==
  note: x = -2.1794 + 0.02953 .*Tc-9.1837 .*(10.^-5) .*(Tc.^2) + 1.4454 .*(10.^-7) .*(Tc.^3);
  Temperature/C : Inport
  -1 : Constant  Value=-7
  -2 : Constant  Value=3
  -5 : Constant  Value=-5
  0.02953 : Constant  Value=0.02953
  0.1 : Constant  Value=9.1837
  0.2 : Constant  Value=1.4454
  Add : Sum  Inputs=+++-
  Constant4 : Constant  Value=-2.1794
  Dashboard Scope : Subsystem  DialogController=hmiCreateDDGDialog  IsWebBlock=on  mask(MathWorksWebBlock){webBlockId=75a5c32c-eec0-415c-91e1-99486c1b84a0, webBlockType=sdiscope, ShowInitialText=on, HMISrcModelName=[]}
      mask prompts: webBlockId "WebBlock Id"; webBlockType "WebBlock Type"; HMISrcModelName "Source Model"
      mask Help: helpview([docroot '/mapfiles/simulink.map'], 'hmi_scope')
      mask Display:
      | if strcmp(get_param(bdroot(gcb),'BlockDiagramType'), 'library')
      |     image([(matlabroot) '/toolbox/simulink/hmi/icons/DashboardScope.png']);
      | end
  Math Function4 : Math  Operator=10^u  SaturateOnIntegerOverflow=on
  Math Function5 : Math  Operator=square  SaturateOnIntegerOverflow=on
  Math Function6 : Math  Operator=10^u  SaturateOnIntegerOverflow=on
  Math Function7 : Math  Operator=pow  SaturateOnIntegerOverflow=on
  Product1 : Product  Inputs=3
  Product2 : Product
  Product3 : Product  Inputs=3
  "water  pressure " : Math  Operator=10^u  SaturateOnIntegerOverflow=on
  Water Pressure : Outport
  wires:
  Add/1 -> "water  pressure "/1
  0.2/1 -> Product3/1
  Math Function7/1 -> Product3/3
  "water  pressure "/1 -> Water Pressure/1  "Water Pressure(atm)"
  0.02953/1 -> Product2/1
  0.1/1 -> Product1/1
  -5/1 -> Math Function4/1
  Math Function4/1 -> Product1/2
  -1/1 -> Math Function6/1
  Temperature/C/1 -> Product2/2, Math Function5/1, Math Function7/1
  Math Function5/1 -> Product1/3
  -2/1 -> Math Function7/2
  Product2/1 -> Add/2
  Product3/1 -> Add/3
  Math Function6/1 -> Product3/2
  Constant4/1 -> Add/1
  Product1/1 -> Add/4

== system Model_FC_v4/Fuel Cell Model/Nernest Voltage (V)/Nernest Voltage/Dashboard Scope ==

== system Model_FC_v4/Fuel Cell Model/Nernest Voltage (V)/Nernest Voltage/If Action Subsystem ==
  In1 : Inport
  Action Port : ActionPort  ActionType=then
  Out1 : Outport
  wires:
  In1/1 -> Out1/1

== system Model_FC_v4/Fuel Cell Model/Nernest Voltage (V)/Nernest Voltage/If Action Subsystem1 ==
  In1 : Inport
  Action Port : ActionPort  ActionType=else
  Out1 : Outport
  wires:
  In1/1 -> Out1/1

== system Model_FC_v4/Fuel Cell Model/Resistance/Activation Overvoltage/Dashboard Scope ==

== system Model_FC_v4/Fuel Cell Model/Resistance/Concentration Overvoltage/Dashboard Scope ==

== system Model_FC_v4/Fuel Cell Model/Resistance/Concentration Overvoltage/If Action Subsystem ==
  In1 : Inport
  Action Port : ActionPort  ActionType=then
  Math Function1 : Math  Operator=log  OutputSignalType=real  SaturateOnIntegerOverflow=on
  Out1 : Outport
  wires:
  In1/1 -> Math Function1/1
  Math Function1/1 -> Out1/1

== system Model_FC_v4/Fuel Cell Model/Resistance/Concentration Overvoltage/If Action Subsystem1 ==
  Action Port : ActionPort  ActionType=else
  Constant1 : Constant  Value=0
  Out1 : Outport
  wires:
  Constant1/1 -> Out1/1

== system Model_FC_v4/Fuel Cell Model/Resistance/Ohmic Overvoltage/Dashboard Scope ==

== system Model_FC_v4/Fuel Cell Model/Nernest Voltage (V)/From Pressure To Partial Pressures/Hydrogen Partial Pressure Output/Dashboard Scope ==

== system Model_FC_v4/Fuel Cell Model/Nernest Voltage (V)/From Pressure To Partial Pressures/Oxygen Partial Pressure Output/Dashboard Scope ==

== system Model_FC_v4/Fuel Cell Model/Nernest Voltage (V)/From Pressure To Partial Pressures/Water Pressure output/Dashboard Scope ==
